simulink model "iPendulumML_Lqr"  (R2017b)
settings: Solver=ode23s  StartTime=0.0  StopTime=10  MaxStep=0.12  RelTol=1e-3
values from neighbouring files (symbols this model uses):
  C = [1, 0, 0;       0, 0, 1]    [iPendelModelParameters.m]
  dphi0 = 1000    [iPendelModelParameters.m]
  dtheta0 = -pi/4    (= -0.785398163397)    [iPendelModelParameters.m]
  g = 9.81    [iPendelModelParameters.m]
  I = Ib + mb*lb^2 + mw*lw^2    (= 0.00102124264)    [iPendelModelParameters.m]
  Iw = 4.20e-5    (= 4.2e-05)    [iPendelModelParameters.m]
  M = mb*lb + mw*lw    (= 0.0146256)    [iPendelModelParameters.m]
  theta0 = pi/4    (= 0.785398163397)    [iPendelModelParameters.m]
undefined symbols (not defined in the file or in its folder): dx0, K_lqr, u_dist
settings Model: Creator=Chris  LastModifiedBy=Georg
settings CodeAppCC: StateflowObjectComments=on

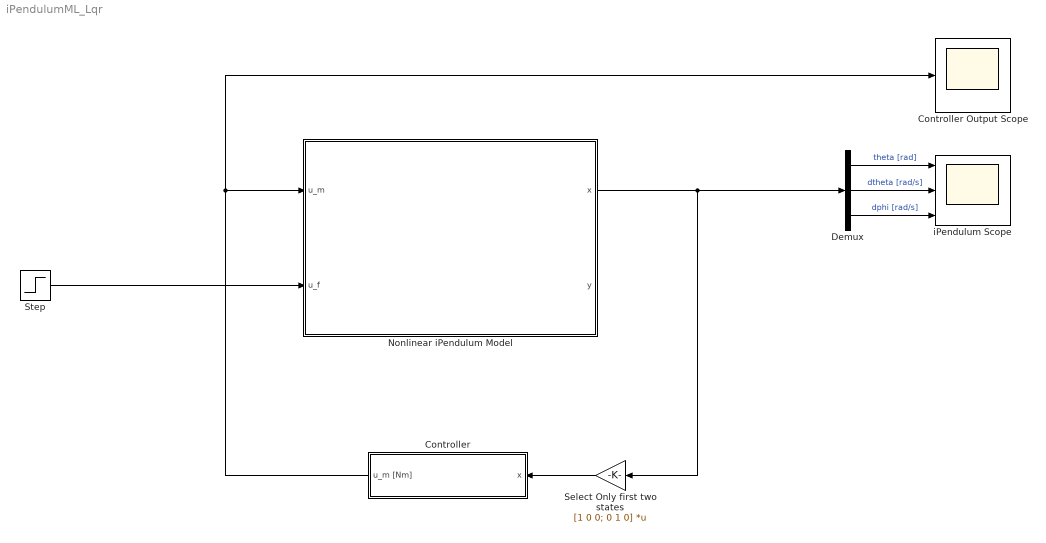
== system iPendulumML_Lqr ==
  Controller : Subsystem
  Controller Output Scope : Scope
  Demux : Demux  Outputs=3
  Nonlinear iPendulum Model : Subsystem
      mask Display:
      | plot([-4 0 4 -4],[4 0 4 4])
      | patch(0+[sin(0), sin(pi* 1/12), sin(pi* 2/12), sin(pi* 3/12), sin(pi* 4/12), sin(pi* 5/12), sin(pi* 6/12), sin(pi* 7/12), sin(pi* 8/12), sin(pi* 9/12), sin(pi* 10/12), sin(pi* 11/12), sin(pi* 12/12), sin(pi* 13/12), sin(pi* 14/12), sin(pi* 15/12), sin(pi* 16/12), sin(pi* 17/12), sin(pi* 18/12), sin(pi* 19/12), sin(pi* 20/12), sin(pi* 21/12), sin(pi* 22/12), sin(pi* 23/12)]*1,2+[cos(0), cos(pi* 1/12), cos(pi* 2/12), cos(pi* 3/12), cos(pi* 4/12), cos(pi* 5/12), cos(pi* 6/12), cos(pi* 7/12), cos(pi* 8/12), cos(pi* 9/12), cos(pi* 10/12), cos(pi* 11/12), cos(pi* 12/12), cos(pi* 13/12), cos(pi* 14/12), cos(pi* 15/12), cos(pi* 16/12), cos(pi* 17/12), cos(pi* 18/12), cos(pi* 19/12), cos(pi* 20/12), cos(pi* 21/12), cos(pi* 22/12), cos(pi* 23/12)]*1)
      | text(-7, 7, '')
      | text( 7, 7, '')
      | text( 0, -2, '')
      | text(-3, 5, 'Nonlinear\n Model')
      | port_label('output', 1, 'x = [theta, dtheta, dphi]') %
      | port_label('output', 2, 'y = [theta, dphi]') %
      | port_label('input',  1, 'u_m [Nm]')
      | port_label('input',  2, 'u_f [Nm]')
  Select Only first two states : Gain  Gain=[1 0 0; 0 1 0]  Multiplication=Matrix(K*u)
  Step : Step  Time=5  After=u_dist  SampleTime=0
  iPendulum Scope : Scope  NumInputPorts=3
  wires:
  Demux/2 -> iPendulum Scope/2  "dtheta [rad/s]"
  Demux/1 -> iPendulum Scope/1  "theta [rad]"
  Demux/3 -> iPendulum Scope/3  "dphi [rad/s]"
  Step/1 -> Nonlinear iPendulum Model/2(u_f)
  Controller/1(u_m [Nm]) -> Nonlinear iPendulum Model/1(u_m), Controller Output Scope/1
  Nonlinear iPendulum Model/1(x) -> Select Only first two states/1, Demux/1
  Select Only first two states/1 -> Controller/1(x)

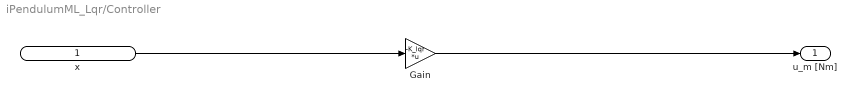
== system iPendulumML_Lqr/Controller ==
  x : Inport
  Gain : Gain  Gain=-K_lqr  Multiplication=Matrix(K*u)
  u_m [Nm] : Outport
  wires:
  x/1 -> Gain/1
  Gain/1 -> u_m [Nm]/1

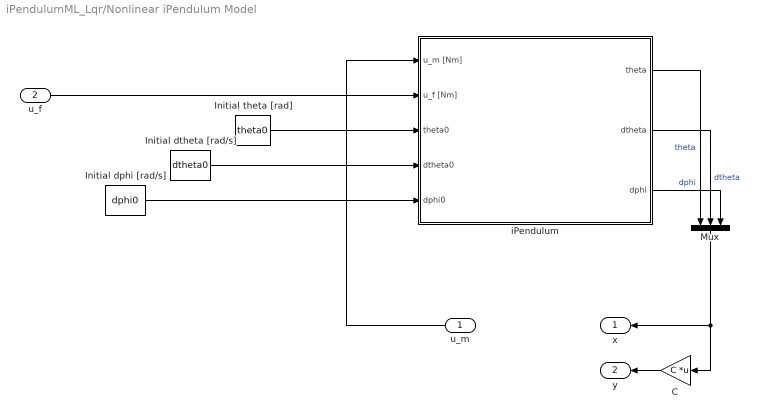
== system iPendulumML_Lqr/Nonlinear iPendulum Model ==
  u_m : Inport
  u_f : Inport  Port=2
  C : Gain  Gain=C  Multiplication=Matrix(K*u) (u vector)
  Initial dphi [rad/s] : Constant  Value=dphi0
  Initial dtheta [rad/s] : Constant  Value=dtheta0
  Initial theta [rad] : Constant  Value=theta0
  Mux : Mux  Inputs=3
  iPendulum : Subsystem
      mask Display:
      | plot([-4 0 4 -4],[4 0 4 4])
      | patch(0+[sin(0), sin(pi* 1/12), sin(pi* 2/12), sin(pi* 3/12), sin(pi* 4/12), sin(pi* 5/12), sin(pi* 6/12), sin(pi* 7/12), sin(pi* 8/12), sin(pi* 9/12), sin(pi* 10/12), sin(pi* 11/12), sin(pi* 12/12), sin(pi* 13/12), sin(pi* 14/12), sin(pi* 15/12), sin(pi* 16/12), sin(pi* 17/12), sin(pi* 18/12), sin(pi* 19/12), sin(pi* 20/12), sin(pi* 21/12), sin(pi* 22/12), sin(pi* 23/12)]*1,2+[cos(0), cos(pi* 1/12), cos(pi* 2/12), cos(pi* 3/12), cos(pi* 4/12), cos(pi* 5/12), cos(pi* 6/12), cos(pi* 7/12), cos(pi* 8/12), cos(pi* 9/12), cos(pi* 10/12), cos(pi* 11/12), cos(pi* 12/12), cos(pi* 13/12), cos(pi* 14/12), cos(pi* 15/12), cos(pi* 16/12), cos(pi* 17/12), cos(pi* 18/12), cos(pi* 19/12), cos(pi* 20/12), cos(pi* 21/12), cos(pi* 22/12), cos(pi* 23/12)]*1)
      | text(-7, 7, '')
      | text( 7, 7, '')
      | text( 0, -2, '')
      | text(-3, 5, 'Nonlinear\n Model')
      | port_label('output', 1, 'theta [rad]')
      | port_label('output', 2, 'dtheta [rad/s]')
      | port_label('output', 3, 'dphi [rad/s]')
      | port_label('input',  1, 'u_m [Nm]')
      | port_label('input',  2, 'u_f [Nm]')
      | port_label('input',  3, 'theta0 [rad]')
      | port_label('input',  4, 'dtheta0 [rad/s]')
      | port_label('input',  5, 'dphi0 [rad/s]')
  x : Outport
  y : Outport  Port=2
  wires:
  C/1 -> y/1
  iPendulum/1(theta) -> Mux/1  "theta"
  u_m/1 -> iPendulum/1(u_m [Nm])
  Mux/1 -> x/1, C/1
  u_f/1 -> iPendulum/2(u_f [Nm])
  Initial dtheta [rad/s]/1 -> iPendulum/4(dtheta0)
  Initial dphi [rad/s]/1 -> iPendulum/5(dphi0)
  Initial theta [rad]/1 -> iPendulum/3(theta0)
  iPendulum/2(dtheta) -> Mux/2  "dtheta"
  iPendulum/3(dphi) -> Mux/3  "dphi"

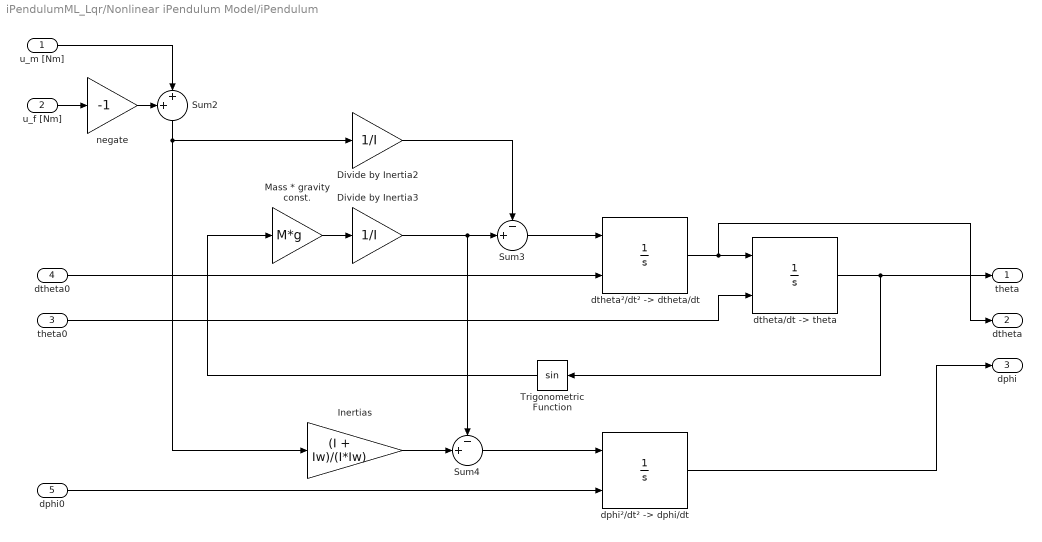
== system iPendulumML_Lqr/Nonlinear iPendulum Model/iPendulum ==
  u_m [Nm] : Inport
  u_f [Nm] : Inport  Port=2
  theta0 : Inport  Port=3
  dtheta0 : Inport  Port=4
  dphi0 : Inport  Port=5
  Divide by Inertia2 : Gain  Gain=1/I
  Divide by Inertia3 : Gain  Gain=1/I
  Inertias : Gain  Gain=(I + Iw)/(I*Iw)
  Mass * gravity const. : Gain  Gain=M*g
  Sum2 : Sum  Inputs=++|
  Sum3 : Sum  Inputs=-+|
  Sum4 : Sum  Inputs=-+|
  Trigonometric Function : Trigonometry
  "dphi²/dt² -> dphi/dt" : Integrator  InitialConditionSource=external  InitialCondition=[dx0, dphi0]
  "dtheta/dt -> theta" : Integrator  InitialConditionSource=external  InitialCondition=[dx0, dphi0]
  "dtheta²/dt² -> dtheta/dt" : Integrator  InitialConditionSource=external  InitialCondition=[dx0, dphi0]
  negate : Gain  Gain=-1
  theta : Outport
  dtheta : Outport  Port=2
  dphi : Outport  Port=3
  wires:
  "dtheta²/dt² -> dtheta/dt"/1 -> "dtheta/dt -> theta"/1, dtheta/1
  u_f [Nm]/1 -> negate/1
  u_m [Nm]/1 -> Sum2/2
  dtheta0/1 -> "dtheta²/dt² -> dtheta/dt"/2
  Divide by Inertia3/1 -> Sum3/2, Sum4/1
  Sum4/1 -> "dphi²/dt² -> dphi/dt"/1
  negate/1 -> Sum2/1
  "dtheta/dt -> theta"/1 -> Trigonometric Function/1, theta/1
  Trigonometric Function/1 -> Mass * gravity const./1
  Sum3/1 -> "dtheta²/dt² -> dtheta/dt"/1
  "dphi²/dt² -> dphi/dt"/1 -> dphi/1
  Mass * gravity const./1 -> Divide by Inertia3/1
  theta0/1 -> "dtheta/dt -> theta"/2
  dphi0/1 -> "dphi²/dt² -> dphi/dt"/2
  Divide by Inertia2/1 -> Sum3/1
  Inertias/1 -> Sum4/2
  Sum2/1 -> Divide by Inertia2/1, Inertias/1
